simulink model "human_lung_R2019b"  (R2019b)
settings: Solver=VariableStepAuto  StartTime=0.0  StopTime=30  RelTol=1e-3
libraries: dspbuff3 x1
settings Model: Creator=upattacini  LastModifiedBy=upattacini
settings SolverCC: ZeroCrossAlgorithm=Adaptive
settings DataIOCC: SaveOutput=off  DSMLogging=off  SaveTime=off  ReturnWorkspaceOutputs=off
settings DebuggingCC: IgnoredZcDiagnostic=none

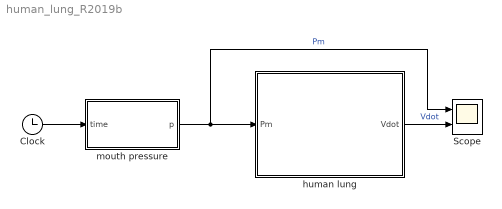
== system human_lung_R2019b ==
  Clock : Clock
  Scope : Scope  NumInputPorts=2
  human lung : Subsystem  mask(Human Lung){E=2.37, R0=0.47, Kv=-0.45, Kf=0.01, K1=0.83, tau1=0.26, tau2=3.89, Ts=0.01, N=32, d=0.01}
      mask prompts: E "E (total lung elasticity) [kPa/l]"; R0 "R0 (airways static resistance) [kPas/l]"; Kv "Kv (volume resistance coefficient) [kPas/l^2]"; Kf "Kf (flow resistance coefficient) [kPas^2/l^2]"; K1 "K1 (viscosity ratio) [−]"; tau1 "tau1 (lung elasticity time constant) [s]"; tau2 "tau2 (lung viscosity time constant) [s]"; Ts "Sample time [s]"; N "Max buffer length"; d "Max deviation threshold"
      mask help: Human Lung
      mask DialogControl Container2 Prompt: Lung Parameters
      mask DialogControl Container3 Prompt: Derivative computation
      mask DialogControl AlgoName Prompt: Adaptive Windows Polynomial Least-Squares Estimator
      mask DialogControl AlgoDescription Prompt: The parameter N identifies the maximum window length for buffering the data. Therefore, the window on which the least-squares algorithm operates on will automatically adapts its length from a minimum of 2 to a maximum of N samples. The greater is N, the more filtered is the derivative. The parameter d allows specifying the maximum deviation threshold for the algorithm. During the validation phase, indeed, the window's length is considered valid if all the computed values from the linear regressor lie within this threshold wrt their corresponding sample values. If not, the window's length is reduced by one step. At each instance, a trial on a window's length enlarged by one step is performed. Therefore, iteration by iteration, the window's length can be adapted by only one step change.
      mask Display: image('assets/lung.png');
  mouth pressure : MATLAB Function  TreatAsAtomicUnit=on
  wires:
  human lung/1(Vdot) -> Scope/2  "Vdot"
  Clock/1 -> mouth pressure/1(time)
  mouth pressure/1(p) -> Scope/1, human lung/1(Pm)  "Pm"

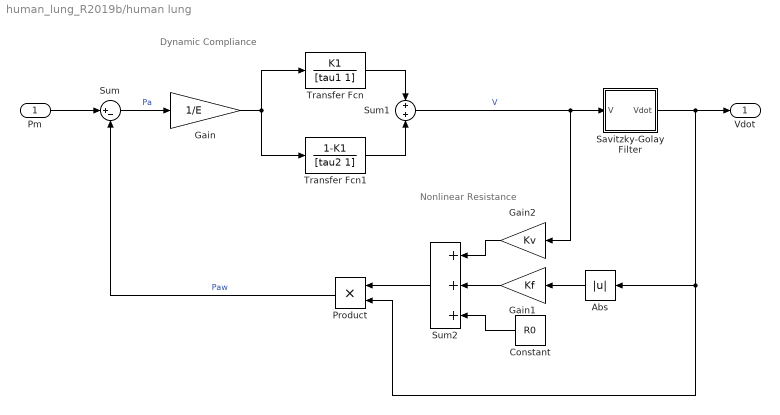
== system human_lung_R2019b/human lung ==
  note: Nonlinear Resistance
  note: Dynamic Compliance
  Pm : Inport
  Abs : Abs
  Constant : Constant  Value=R0
  Gain : Gain  Gain=1/E
  Gain1 : Gain  Gain=Kf
  Gain2 : Gain  Gain=Kv
  Product : Product
  Savitzky-Golay Filter : Subsystem  mask{Ts=Ts, N=N, d=d}
      mask prompts: Ts "Sample time [s]"; N "Max buffer length"; d "Max deviation threshold"
      mask Display: disp('du/dt', 'texmode','on');
  Sum : Sum  Inputs=|+-
  Sum1 : Sum
  Sum2 : Sum  Inputs=3
  Transfer Fcn : TransferFcn  Numerator=K1  Denominator=[tau1 1]
  Transfer Fcn1 : TransferFcn  Numerator=1-K1  Denominator=[tau2 1]
  Vdot : Outport
  wires:
  Gain/1 -> Transfer Fcn1/1, Transfer Fcn/1
  Transfer Fcn/1 -> Sum1/1
  Sum/1 -> Gain/1  "Pa"
  Transfer Fcn1/1 -> Sum1/2
  Sum1/1 -> Savitzky-Golay Filter/1(V), Gain2/1  "V"
  Pm/1 -> Sum/1
  Abs/1 -> Gain1/1
  Gain2/1 -> Sum2/1
  Gain1/1 -> Sum2/2
  Constant/1 -> Sum2/3
  Product/1 -> Sum/2  "Paw"
  Sum2/1 -> Product/1
  Savitzky-Golay Filter/1(Vdot) -> Vdot/1, Abs/1, Product/2

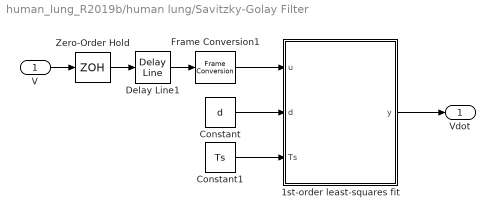
== system human_lung_R2019b/human lung/Savitzky-Golay Filter ==
  V : Inport
  1st-order least-squares fit : MATLAB Function  TreatAsAtomicUnit=on
  Constant : Constant  Value=d
  Constant1 : Constant  Value=Ts
  Delay Line1 : dspbuff3/Delay Line  siz=N  ic=0  directfeed=off  enable_output=off  hold_output=off  OutputFrames=on
      settings: SourceProductBaseCode=DS
  Frame Conversion1 : FrameConversion  OutFrame=Sample-based
  Zero-Order Hold : ZeroOrderHold  SampleTime=Ts
  Vdot : Outport
  wires:
  Delay Line1/1 -> Frame Conversion1/1
  Frame Conversion1/1 -> 1st-order least-squares fit/1(u)
  1st-order least-squares fit/1(y) -> Vdot/1
  V/1 -> Zero-Order Hold/1
  Constant/1 -> 1st-order least-squares fit/2(d)
  Constant1/1 -> 1st-order least-squares fit/3(Ts)
  Zero-Order Hold/1 -> Delay Line1/1

== matlab function human_lung_R2019b/mouth pressure ==
  data: time input; p output
function p = mouth_pressure(time)

pip = 0.85;

t = mod(time, 7);
if t < 2
    p = 1 - exp(-t/0.4);
elseif t < 3
    p = pip;
else
    t = t - 3;
    p = pip * exp(-t/0.2);
end

== matlab function human_lung_R2019b/human lung/Savitzky-Golay Filter/1st-order least-squares fit ==
  data: u input; y output; d input; Ts input
function y=savitzky_golay_filter(u,d,Ts)
% Adaptive Window Polynomial Fitting Estimator
% https://doi.org/10.1109/87.880606
%#ok<*NASGU>

coder.extrinsic('polyfit_helper');

persistent n;
if isempty(n)
    n=1;
end

L=length(u);
pos=zeros(1,2);
Ly=0;
N=n;

for j=max(1,n-1):min(n+1,L-1)
    pos=polyfit_helper(u,1,Ts,j);

    finish=false;
    for i=0:j
        Ly=polyval(pos,i*Ts);
        if abs(u(L-j+i)-Ly)>d
            finish=true;
            break;
        end
    end
    
    if finish
        N=j;
        break;
    end
    N=j;
end

y=pos(1);
n=N;
